simulink model "KITTDynamicsFinal"  (R2015b)
settings: Solver=FixedStepAuto  StartTime=0.0  StopTime=8  FixedStep=0.01  RelTol=1e-3
values from neighbouring files (symbols this model uses):
  b = 0.0015    [KITTParameters.m]
  c = 0.02    [KITTParameters.m]    (also in directionkeys.m = 0)
  Fin = -120    [KITTDynamicsRun.m]
  m = 13    [KITTParameters.m]
  Vi = 60/3.6    (= 16.6666666667)    [KITTDynamicsRun.m]
undefined symbols (not defined in the file or in its folder): magnitude
settings Model: Creator=koenm  LastModifiedBy=koenm
settings DataIOCC: SaveFormat=StructureWithTime
settings DebuggingCC: AlgebraicLoopMsg=none

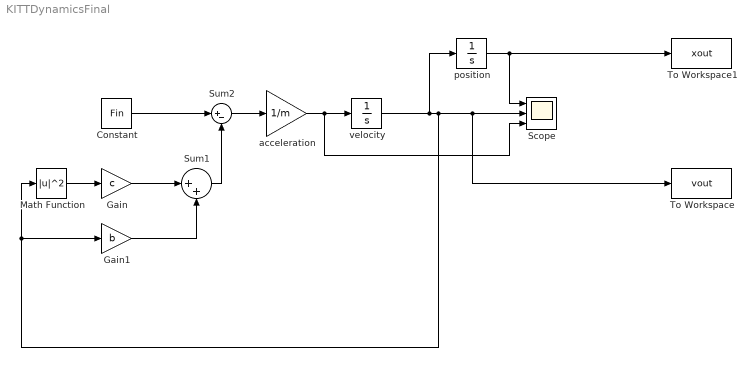
== system KITTDynamicsFinal ==
  Constant : Constant  Value=Fin
  Gain : Gain  Gain=c
  Gain1 : Gain  Gain=b
  Math Function : Math  Operator=magnitude^2  SaturateOnIntegerOverflow=on
  Scope : Scope  NumInputPorts=3
  Sum1 : Sum  Inputs=|++
  Sum2 : Sum  Inputs=|+-
  To Workspace : ToWorkspace  VariableName=vout  SaveFormat=Timeseries  SampleTime=-1
  To Workspace1 : ToWorkspace  VariableName=xout  SaveFormat=Timeseries  SampleTime=-1
  acceleration : Gain  Gain=1/m
  position : Integrator
  velocity : Integrator  InitialCondition=Vi
  wires:
  Math Function/1 -> Gain/1
  Gain/1 -> Sum1/1
  Gain1/1 -> Sum1/2
  position/1 -> Scope/1, To Workspace1/1
  Sum1/1 -> Sum2/2
  velocity/1 -> position/1, Gain1/1, Math Function/1, To Workspace/1, Scope/2
  Constant/1 -> Sum2/1
  Sum2/1 -> acceleration/1
  acceleration/1 -> Scope/3, velocity/1
